simulink model "kessel_loch_pi_modell"  (R2024a)
settings: Solver=VariableStepAuto  StartTime=0.0  StopTime=20  RelTol=1e-3
undefined symbols (not defined in the file or in its folder): TN
settings Model: Creator=janho  LastModifiedBy=janho

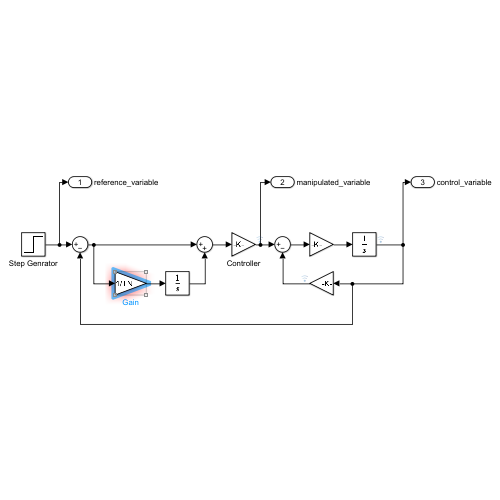
[thumbnail: Simulink's stored preview of the top-level diagram]
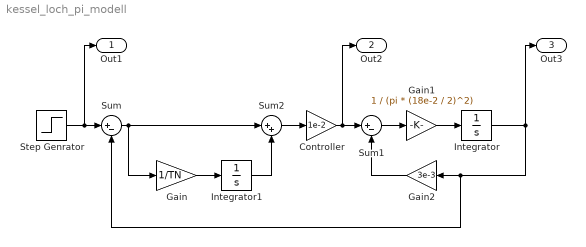
== system kessel_loch_pi_modell ==
  Controller : Gain  Gain=1e-2
  Gain : Gain  Gain=1/TN
  Gain1 : Gain  Gain=1 / (pi * (18e-2 / 2)^2)
  Gain2 : Gain  Gain=3e-3
  Integrator : Integrator
  Integrator1 : Integrator
  Step Genrator : Step  Time=0  After=10e-2  SampleTime=0
  Sum : Sum  Inputs=|+-
  Sum1 : Sum  Inputs=|+-
  Sum2 : Sum  Inputs=|++
  Out1 : Outport  SignalName=reference_variable
  Out2 : Outport  Port=2  SignalName=manipulated_variable
  Out3 : Outport  Port=3  SignalName=control_variable
  wires:
  Integrator/1 -> Out3/1, Sum/2, Gain2/1
  Gain2/1 -> Sum1/2
  Sum/1 -> Sum2/1, Gain/1
  Step Genrator/1 -> Out1/1, Sum/1
  Sum1/1 -> Gain1/1
  Gain1/1 -> Integrator/1
  Gain/1 -> Integrator1/1
  Integrator1/1 -> Sum2/2
  Sum2/1 -> Controller/1
  Controller/1 -> Out2/1, Sum1/1
